simulink model "wtLinModelSimulink"  (R2021b)
settings: Solver=VariableStepAuto  StartTime=0.0  StopTime=10.0  RelTol=1e-3
values from neighbouring files (symbols this model uses):
  u_op = [simulationData(1,senIdx.Vhfree); simulationData(1,senIdx.pnt413); simulationData(1,senIdx.pfo017)]    [wtLin_V164_8MW_V6_LQI.m]
  x_init = x_op_temp_flc + x_bar_init_flc    [wtLin_V164_8MW_V6_LQI.m]
undefined symbols (not defined in the file or in its folder): A, B, C, x_op
settings Model: Creator=martin  LastModifiedBy=martin

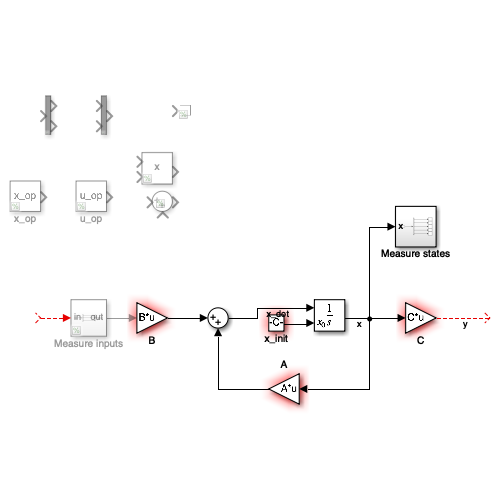
[thumbnail: Simulink's stored preview of the top-level diagram]
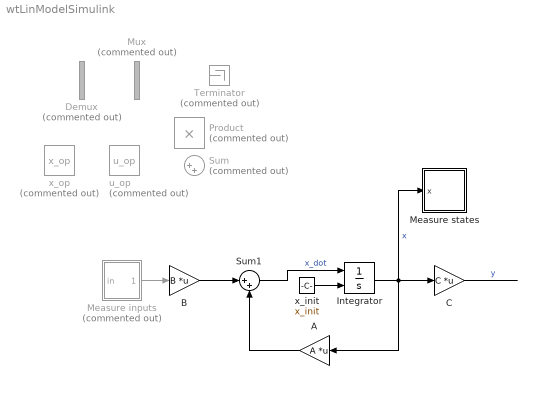
== system wtLinModelSimulink ==
  A : Gain  Gain=A  Multiplication=Matrix(K*u)
  B : Gain  Gain=B  Multiplication=Matrix(K*u)
  C : Gain  Gain=C  Multiplication=Matrix(K*u)
  Demux : Demux  Commented=on  Outputs=2
  Integrator : Integrator  InitialConditionSource=external
  Measure inputs : Subsystem  Commented=on
  Measure states : Subsystem
  Mux : Mux  Commented=on  Inputs=2
  Product : Product  Commented=on
  Sum : Sum  Commented=on  Inputs=|++
  Sum1 : Sum  Inputs=|++
  Terminator : Terminator  Commented=on
  u_op : Constant  Commented=on  Value=u_op
  x_init : Constant  Value=x_init
  x_op : Constant  Commented=on  Value=x_op
  wires:
  A/1 -> Sum1/2
  Sum1/1 -> Integrator/1  "x_dot"
  B/1 -> Sum1/1
  ? -> Measure inputs/1(in)
  x_init/1 -> Integrator/2
  Integrator/1 -> C/1, Measure states/1(x), A/1  "x"
  Measure inputs/1(out) -> B/1
  C/1 -> ?  "y"

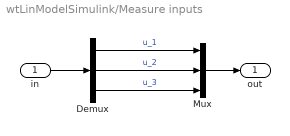
== system wtLinModelSimulink/Measure inputs ==
  in : Inport
  Demux : Demux  Outputs=3
  Mux : Mux  Inputs=3
  out : Outport
  wires:
  Demux/1 -> Mux/1  "u_1"
  Demux/2 -> Mux/2  "u_2"
  Demux/3 -> Mux/3  "u_3"
  Mux/1 -> out/1
  in/1 -> Demux/1

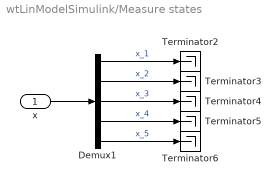
== system wtLinModelSimulink/Measure states ==
  x : Inport
  Demux1 : Demux  Outputs=5
  Terminator{2..6} (5 alike) : Terminator
  wires:
  Demux1/5 -> Terminator6/1  "x_5"
  Demux1/3 -> Terminator4/1  "x_3"
  Demux1/1 -> Terminator2/1  "x_1"
  Demux1/2 -> Terminator3/1  "x_2"
  Demux1/4 -> Terminator5/1  "x_4"
  x/1 -> Demux1/1
